simulink model "day10p2"  (R2026a)
settings: Solver=FixedStepDiscrete  StopTime=inf
InitFcn:
  | % lmpCntMax = 6;
  | lmpCntMax = 10;
  | % btnCntMax = 10;
  | btnCntMax = 16;
  | % btnStrMax = 39;
  | btnStrMax = 181;
  | % jltStrMax = 17;
  | jltStrMax = 39;
  | lmpStrMax = lmpCntMax + 2;
  | possibilities = dec2bin([0:((2^btnCntMax) - 1)]) - '0';
  | [~, ixs] = sort(sum(possibilities, 2));
  | possibilities = possibilities(ixs, :);
undefined symbols (not defined in the file): DiscIntNeverNeededParam
libraries: simulink x12
(part 1 of 2)
settings Model: PauseTimes=14  Creator=pete  LastModifiedBy=pete

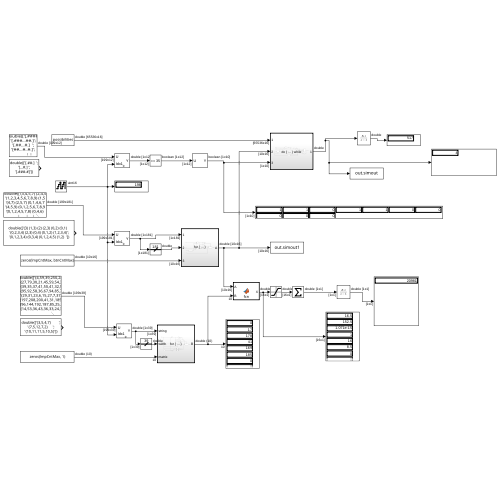
[thumbnail: Simulink's stored preview of the top-level diagram]
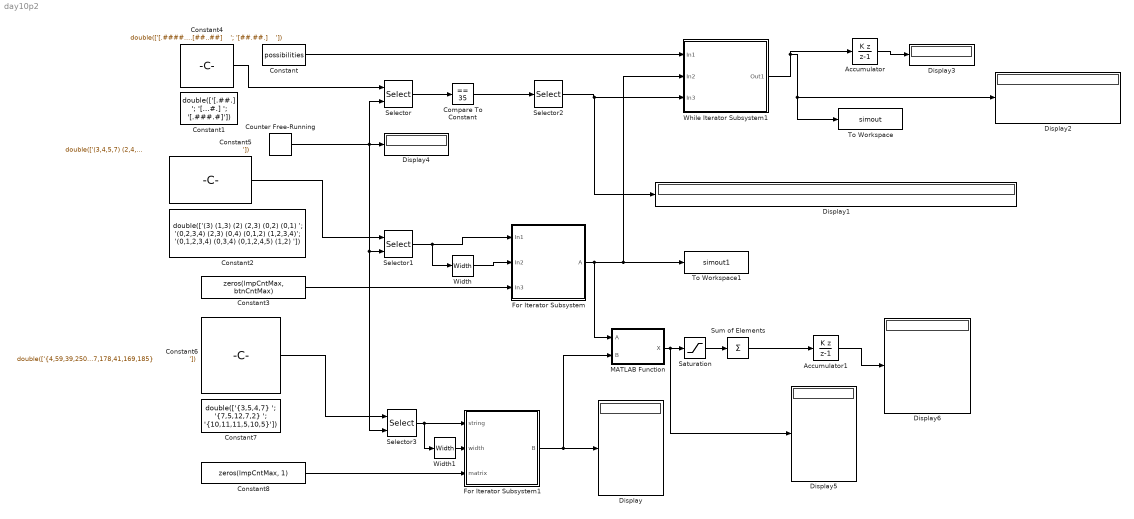
== system day10p2 ==
  Accumulator : DiscreteIntegrator  IntegratorMethod=Accumulation: Backward Euler  SampleTime=-1  ICPrevOutput=DiscIntNeverNeededParam  ICPrevScaledInput=DiscIntNeverNeededParam
  Accumulator1 : DiscreteIntegrator  IntegratorMethod=Accumulation: Backward Euler  SampleTime=-1  ICPrevOutput=DiscIntNeverNeededParam  ICPrevScaledInput=DiscIntNeverNeededParam
  Compare To Constant : simulink/Logic and Bit Operations/Compare To Constant  relop===  const=35  OutDataTypeStr=boolean
  Constant : Constant  Value=possibilities
  Constant1 : Constant  Value=|
      | double(['[.##.]  ';
      | '[...#.] ';
      | '[.###.#]'])
  Constant2 : Constant  Value=|
      | double(['(3) (1,3) (2) (2,3) (0,2) (0,1)        ';
      | '(0,2,3,4) (2,3) (0,4) (0,1,2) (1,2,3,4)';
      | '(0,1,2,3,4) (0,3,4) (0,1,2,4,5) (1,2)  '])
  Constant3 : Constant  Value=zeros(lmpCntMax, btnCntMax)
  Constant4 : Constant  Value=|
      | double(['[.####.#.]  ';
      | '[.###...##.]';
      | '[.##...#.]  ';
      | '[##...#..#.]';
      | '[#...#.#..] ';
      | '[.##...]    ';
      | '[###.....#] ';
      | '[.#.#....]  ';
      | '[###..#..#] ';
      | '[.###]      ';
      | '[...#..#.]  ';
      | '[#.##]      ';
      | '[#####.##.] ';
      | '[.#####]    ';
      | '[.#..###]   ';
      | '[...##.]    ';
      | '[#####.]    ';
      | '[#.##.]     ';
      | '[#....#.##] ';
      | '[.#.#]      ';
      | '[#.#.##.##.]';
      | '[...#]      ';
      | '[..##.#]    ';
      | '[#####.]    ';
      | '[#...#.#]   ';
      | '[##.#..]    ';
      | '[.#..#]     ';
      | '[###.]      ';
      | '[##..#.#..] ';
      | '[###.]      ';
      | '[###.]      ';
      | '[.###]      ';
      | '[##...#.]   ';
      | '[.###.#.]   ';
      | '[#.#...]    ';
      | '[#..##.]    ';
      | '[..##...]   ';
      | '[..#...#]   ';
      | '[.#...##]   ';
      | '[..#..#.#]  ';
      | '[###......] ';
      | '[#.####.]   ';
      | '[..##.##]   ';
      | '[.###]      ';
      | '[.##.#.#..] ';
      | '[#.#.]      ';
      | '[###..#.#]  ';
      | '[#.#..#.]   ';
      | '[#...##]    ';
      | '[...###..]  ';
      | '[####.]     ';
      | '[#...####]  ';
      | '[##.##....#]';
      | '[.#..#]     ';
      | '[#...#....] ';
      | '[.#.....###]';
      | '[..#.#..#]  ';
      | '[#.##..]    ';
      | '[..##...##] ';
      | '[#.#.....#] ';
      | '[.#..##]    ';
      | '[..###]     ';
      | '[.#....#.]  ';
      | '[#.#....###]';
      | '[...#.#.#.] ';
      | '[#..##]     ';
      | '[####]      ';
      | '[..#...##]  ';
      | '[#..#]      ';
      | '[.####.]    ';
      | '[..##.#..##]';
      | '[#.#..##]   ';
      | '[...#..#.]  ';
      | '[#.##...#..]';
      | '[.#..####.#]';
      | '[.#.#]      ';
      | '[##..#.###] ';
      | '[.##.....#.]';
      | '[.....#.#]  ';
      | '[#.#.]      ';
      | '[#.####.###]';
      | '[.##.]      ';
      | '[###..]     ';
      | '[##...#.]   ';
      | '[.#.#.#]    ';
      | '[#...##.]   ';
      | '[###.]      ';
      | '[...#]      ';
      | '[#...#..]   ';
      | '[##..#]     ';
      | '[...#]      ';
      | '[###.]      ';
      | '[#..#####.] ';
      | '[#.#.]      ';
      | '[#...]      ';
      | '[#..##.]    ';
      | '[.#.....]   ';
      | '[###.]      ';
      | '[##...####.]';
      | '[.####.#.#.]';
      | '[.#.##]     ';
      | '[######...] ';
      | '[#..#..#]   ';
      | '[.##...#.]  ';
      | '[...#.#]    ';
      | '[##..#.#.##]';
      | '[....##..]  ';
      | '[####..#.]  ';
      | '[#....#..##]';
      | '[....#]     ';
      | '[.#.#.]     ';
      | '[##...#.#.] ';
      | '[#...#]     ';
      | '[....#]     ';
      | '[###.##..]  ';
      | '[#.#.]      ';
      | '[..#..#]    ';
      | '[#.#.#]     ';
      | '[.#.##]     ';
      | '[.#.#.###..]';
      | '[######..]  ';
      | '[##.##]     ';
      | '[###.##]    ';
      | '[......#..] ';
      | '[##.#.]     ';
      | '[##.#.##..#]';
      | '[.###.]     ';
      | '[..##.###.] ';
      | '[#.#....]   ';
      | '[...#.#..]  ';
      | '[..#.##....]';
      | '[#.##]      ';
      | '[...##]     ';
      | '[#####.#]   ';
      | '[#.##..]    ';
      | '[##..#####] ';
      | '[...##.##.] ';
      | '[.#.#]      ';
      | '[##..]      ';
      | '[.....##..] ';
      | '[###.#..#]  ';
      | '[.##.#.###.]';
      | '[..####]    ';
      | '[#.......##]';
      | '[##.##.]    ';
      | '[###..##]   ';
      | '[####..#.#] ';
      | '[.###..#.#.]';
      | '[.###]      ';
      | '[.....###.#]';
      | '[.###..###.]';
      | '[##.#]      ';
      | '[#.#.]      ';
      | '[.#..#]     ';
      | '[..###]     ';
      | '[.######]   ';
      | '[####...#.] ';
      | '[.#.....#.] ';
      | '[...#.###]  ';
      | '[####]      ';
      | '[#.####..]  ';
      | '[...####]   ';
      | '[#.##.#....]';
      | '[#...###]   ';
      | '[.#.#]      ';
      | '[.##.#.##.] ';
      | '[.##.##.]   ';
      | '[##.#.]     ';
      | '[#.#.]      ';
      | '[#.#.]      ';
      | '[##.###.##.]';
      | '[..##.#.]   ';
      | '[#..##.###.]';
      | '[#......#.] ';
      | '[......#..#]';
      | '[#..#.##]   ';
      | '[...###.]   ';
      | '[..#.#...#.]';
      | '[.#.#.#####]';
      | '[#.#....]   ';
      | '[#.##]      ';
      | '[.#.#.###.#]';
      | '[#.###.]    ';
      | '[#...#.....]';
      | '[.###.##.]  ';
      | '[.....#]    ';
      | '[.####.#..#]';
      | '[.#....]    ';
      | '[.#...]     ';
      | '[#.##.###.#]';
      | '[.###.]     ';
      | '[##.##]     ';
      | '[#.#...##.] ';
      | '[#....##.]  ';
      | '[#.#.###]   ';
      | '[#.##.#..##]';
      | '[##..##.#]  ';
      | '[##..##]    ';
      | '[##.##.]    '])
  Constant5 : Constant  Value=|
      | double(['(3,4,5,7) (2,4,5,6,7) (1,4,7) (1,3,4,7) (1,2,3,4,5,7) (7) (1,2,3,6) (0,1,3,6,7)                                                                                                      ';
      | '(1,2,3,4,5,6,7,8,9) (1,5) (0,1,3,4,5,6,7,8,9) (4,8,9) (0,6,7,9) (1,6,8) (0,1,2,5,6,7,8) (0,1,2,3,5,7,8,9) (1,2,4,5)                                                                  ';
      | '(4,7) (2,5,7) (0,1,4,6,7) (1,4) (0,3,4,5,6,7) (0,1,2,3,4,5,7) (0,1,2,3,4,6) (2,3,5,6,7)                                                                                              ';
      | '(4,5,9) (0,1,2,5,6,7,8,9) (0,1,4,5,6,7,9) (0,1,2,5,6,8) (0,1,2,3,5,7) (1,2,3,4,5,6,8,9) (0,1,3,4,5,6,7,8,9) (3,4,8) (0,4,7,9)                                                        ';
      | '(0,1,2,4,5,7,8) (0,4,6) (0,1,2,7,8) (1,7,8) (1,2,3) (0,5,7,8) (0,1,4,5,6,7) (1,2,5,7,8)                                                                                              ';
      | '(1,3,4) (0,1,3) (3,5) (0) (0,1,2,5) (2,3,4)                                                                                                                                          ';
      | '(0,1,2,3,4,8) (0,3,4,7) (0,1,2,4,5,6,7) (2,3,4) (0,4) (1,2,3,7,8) (0,2,3,6,8) (0,2,4,5,7) (0,1,4,5,6,7,8)                                                                            ';
      | '(1,2,3,4,5,6,7) (1,3) (1,2,3,4,5,7) (1,7) (0,1,2,3,4,6,7) (0,2,4,5,6)                                                                                                                ';
      | '(1,4,5,6) (0,3,7) (1,6,7) (1,2,3,4,8) (0,4,7) (3,4,7) (2,3,5,8)                                                                                                                      ';
      | '(3) (0) (1,3) (1,2) (0,2,3)                                                                                                                                                          ';
      | '(0,2,3,5,6) (1,3,5,6) (5,7) (0,4,7) (1,7) (0,1) (2,4) (0,2,3,4,5,6) (0,3,4,5,6,7) (0)                                                                                                ';
      | '(1,3) (0,3) (0,2,3)                                                                                                                                                                  ';
      | '(1,5,8) (1,2,3,5,6) (2,4,8) (3,4,8) (2,4) (0,1,7,8) (2,3,6) (2,3,7,8) (4,7)                                                                                                          ';
      | '(0,1,3) (0,2) (0,3,4,5) (0,1,4) (0,4)                                                                                                                                                ';
      | '(0,1,4) (1,2) (1,2,3,4,5,6) (0,3,5) (2,3)                                                                                                                                            ';
      | '(2,5) (3) (1,4) (0,1) (0,1,4,5) (4) (2,4,5) (1,2,3,4)                                                                                                                                ';
      | '(0,1,3,4,5) (1,2,3,4) (3) (3,5) (1,5) (0,1,2,4) (2,5) (0,1,2,3)                                                                                                                      ';
      | '(0,1,3,4) (0,1,3) (0,2,3)                                                                                                                                                            ';
      | '(4) (2,3,7) (2,3,4,7,8) (0,1,4,5) (2,3,5,6) (1,2,3,5,6,7,8) (0,3,5,7)                                                                                                                ';
      | '(1,2) (0,2) (0,1,2) (3)                                                                                                                                                              ';
      | '(2,5,6,8) (0,1,2,3,4,5,7,8) (2,7) (0,2,3,6,8) (0,4,6,7,9) (0,1,3,4,5,8,9) (3,4,8) (0,1,5,8)                                                                                          ';
      | '(0,3) (0,2) (1,3) (0,1,3)                                                                                                                                                            ';
      | '(1,3) (0,5) (2,3,4) (0,1,3,4) (1,2,5)                                                                                                                                                ';
      | '(3,4,5) (0,1,2,4,5) (2,3,5) (0,1,5) (1,2,3) (0,2,4,5) (4,5)                                                                                                                          ';
      | '(3,5,6) (0,1,2,5,6) (0,1,2,3,6) (4,6) (2,4,5,6) (0,1,2,3,4) (1,2,3) (0,1,2,4,5) (1,2,3,4,6)                                                                                          ';
      | '(1,2,3,5) (0,3,4,5) (1,2) (0,1,3)                                                                                                                                                    ';
      | '(0,2) (1,4) (0,1,3,4) (0,3,4)                                                                                                                                                        ';
      | '(3) (0) (0,1) (0,1,2) (1,2)                                                                                                                                                          ';
      | '(0,3,4,5,6,7,8) (1,2,4,5,6,7,8) (2,4,7) (0,1,4,6) (1,2,3,4,5,6,7) (1,3,4,5,6) (0,1,3,5,8) (0,1,4,8)                                                                                  ';
      | '(0,1,2) (0,1,3)                                                                                                                                                                      ';
      | '(1,2) (0,2,3) (0,3) (0,1)                                                                                                                                                            ';
      | '(1,2,3) (0,2,3)                                                                                                                                                                      ';
      | '(3,4,6) (1,2,4,5) (0,1,5) (1,6) (0,2,3,5,6)                                                                                                                                          ';
      | '(0,1,2,3,6) (2,3,5,6) (1,2) (3,5) (0,2,4,5,6) (1)                                                                                                                                    ';
      | '(1,4,5) (0,3,4,5) (3,4) (2,5)                                                                                                                                                        ';
      | '(0,1,4,5) (1,2,5) (0,1,2,4) (3,5)                                                                                                                                                    ';
      | '(2,3) (0,1,3,5,6) (2,4) (0,2,3,4,5,6) (0,5)                                                                                                                                          ';
      | '(0,2,6) (1,3) (0,1,2,3,5,6) (1,3,4,5,6) (4,5,6) (1,2,3,4)                                                                                                                            ';
      | '(1,2,4,5) (0,2,3,4,5) (0,2) (0,5) (0,2,4,6) (1,5,6)                                                                                                                                  ';
      | '(1,2,4,7) (1,4,5) (0,1,3,6) (0,1,2,4,6) (2,3,5,7) (0,3,4,5,6,7)                                                                                                                      ';
      | '(0,1,3,4,7) (1,2,3) (1,8) (2,7) (0,1,4,5,7,8) (0,1,3,6,7) (0,1,2,3,4,5,7) (0,1,4,7,8) (0,1,3,4,6,7,8)                                                                                ';
      | '(0,2,3,4,5) (0,1,3,5,6) (0,3,4,5) (0,1,5,6) (2) (1,2,3,4,6) (0,1,3,4,5) (0,1,2,3) (0,6)                                                                                              ';
      | '(2,3) (1,4,5,6) (1,2,3,4,5,6) (0,1,2,5,6) (4,5) (0,1,2,3) (1,4) (0,1,3) (0,5)                                                                                                        ';
      | '(0,1) (2,3) (0,2,3)                                                                                                                                                                  ';
      | '(0,1,4,5,6,7,8) (0,1,3,4,5,6,7) (0,1,2,4,5,7,8) (0,1,2,3,4,6,8) (0,1,3,4,5,7,8) (0,2,3) (5,7)                                                                                        ';
      | '(0,1) (2,3) (1,2) (0,3) (0,2)                                                                                                                                                        ';
      | '(0,1,3,4,6,7) (1,2,3,4,5,7) (0,1,7) (1,4,5,6,7) (0,1,5,7) (5,6,7) (0,4) (1,5) (2,3,4,5) (1,4,7)                                                                                      ';
      | '(1,3,4) (0,1,3) (1,3,4,5,6) (1,2,3,5) (0,2,3,4,5)                                                                                                                                    ';
      | '(0,4,5) (3,4) (0,1,2,3,5) (1,2) (1)                                                                                                                                                  ';
      | '(3,4) (0,2,5,6,7) (0,3,5,6) (0,1,2,3,5,7) (1,2,4,5,7) (0,1,3,4,5) (0,2) (2,6,7) (0,1,4,5,6,7) (2,3,4,5,6,7)                                                                          ';
      | '(4) (0,1,3,4) (2,3,4) (1,2,3) (2) (0,3,4) (2,4)                                                                                                                                      ';
      | '(0,1,3,4) (4,5,6,7) (0,1,2,4,5,6,7) (0) (0,1,2,3,5,7) (0,2,3,7) (1,5) (0,2,3,4,6,7)                                                                                                  ';
      | '(1,5,9) (1,3,5,6,7,8,9) (1,2,4,5,8,9) (1,2,4,5,6,7) (1,3,5,6,7,8) (0,1,2,3,4,5,6,7,9) (0,1,3,4,6,7,8,9) (0,1,5,6,7,9) (2,4,6,7,8)                                                    ';
      | '(0,2,4) (0,2) (0,1,2) (1,4) (2,3,4) (1,2,3,4)                                                                                                                                        ';
      | '(0,1,2,4,8) (0,1,4,5,6,7,8) (3,4,5,6,7,8) (1,3,7,8) (0,2,3,4,8) (2,3) (3,6,7) (0,1,4,5,7) (0,1,5,6) (2,7) (0,6,8)                                                                    ';
      | '(0,1,2,3,5,6,7,8,9) (0,2,3,4,6,7,9) (0,1,2,5,8) (0,1,3,7,8,9) (1,4,5,6,7) (0,1,3,8) (0,1,2,3,5,6,8) (0,1,3,4,5,6,7) (1,2,3,5) (1,3,4,5,6,7,8,9)                                      ';
      | '(0,1,2,3,6) (4,6) (1,2,3,5) (2,3,7) (0,5,6) (0,1,4,6) (0,1,3,5) (1,6,7) (4,7)                                                                                                        ';
      | '(0,1,3,4) (3,4,5) (2,3,4,5) (2,3) (4,5) (1,5)                                                                                                                                        ';
      | '(4,8) (1,4,6,8) (3) (0,1,5) (5,7) (1,2,3,5,7,8) (2,3,4,5) (0) (1,3,4) (0,1,3,4,6,7,8)                                                                                                ';
      | '(6,8) (1,2,3,4,7,8) (1,6,8) (1,2,3,6,7) (1,2,3,5,8) (2,6) (3,4,5,8) (0,2) (1,2,3,4,5,6)                                                                                              ';
      | '(2,4,5) (0,1,3) (4,5) (0,1,5) (0,2,3,4,5)                                                                                                                                            ';
      | '(1,2) (0,1,3) (1,3,4)                                                                                                                                                                ';
      | '(6) (0,4,5) (1,2,4,6) (1,2,3,4,7) (0,1,2,3) (0,1,2,4,5,7) (0,4) (1,7) (0,3,7)                                                                                                        ';
      | '(0,1,2,3,4,5,6,8) (1,3,4,5,7,8,9) (1,2,3,5,6,7,9) (6,8) (6,7) (1,3,5,7,8) (0,1,2,3,6,8,9) (1,2,4,5,6,7,8,9) (0,1,2,3,5,6,8,9) (0,1,4,5,6,7,8,9)                                      ';
      | '(0,1,2,6,7) (0,1,3,4,5,7,8) (1,3,8) (0,1,3,4,6,7,8) (1) (0,2,4,6,7,8) (4) (3,5,7) (0,1,4,8) (1,4,6) (1,2,3,4,7,8)                                                                    ';
      | '(0,1,2,4) (0,3) (0,2,4) (0,2) (1,4)                                                                                                                                                  ';
      | '(0,1,2) (3) (0,3) (0,1,3) (0,1)                                                                                                                                                      ';
      | '(2,3,4,5,6) (0,1,2,3,4,5,7) (0,4,5,6,7) (1,6,7) (0,1,2) (4,5,6,7) (1,3,4,5,6,7)                                                                                                      ';
      | '(0,1) (1,3) (1,2) (3) (0,3) (0,2)                                                                                                                                                    ';
      | '(1,2,4,5) (0,2,3,5) (0,4,5) (0,2)                                                                                                                                                    ';
      | '(2,3,4,5,9) (2,3,4,6,8,9) (0,1,2,3,5,6,7,9) (3,5,6,9) (0,8) (0,3,4,5,6,9) (0,4,8) (1,3,7,8) (1,4,5,7,8) (0,3,4,5) (0,2,3,4,6,7)                                                      ';
      | '(1,2,4,6) (2,5,6) (3,4) (1,3,4,5,6) (0,1,2,4,6) (0,5) (0,1,2,5)                                                                                                                      ';
      | '(1,2,3) (1,4) (0,1,3,4,5,7) (0,7) (1,5) (1,7) (0,2,4,5,6,7) (0,4) (3) (4,5)                                                                                                          ';
      | '(1,2,6,7) (0) (3,4) (0,1,2,5,7,8,9) (7,8) (0,1,2,3,4,6,7,8,9) (6,7,9) (1,2,4,5,7) (0,3,7) (1,3,4,5,6,7,8,9) (1,3,4,6,7,8,9) (0,1,2,4,6)                                              ';
      | '(0,5,7,8) (2,3,4,8,9) (1,2,3,5,8) (0,1,3,4,5,7,8,9) (4,5,6,7,8) (0,2,3,5,8,9) (1,2) (0,1,2,3,6,8) (0,2,4,5,8)                                                                        ';
      | '(1,2) (0,1,3) (2,3)                                                                                                                                                                  ';
      | '(0,2,3,6,7,8) (1,2,5,7) (0,1,2,3,6,7) (2) (0,4,5,8) (1,3,6,7,8) (1,4,5,7,8) (0,2,4,5,6,7) (0,1,2,4,6,7,8) (1,3,5) (1,4,6)                                                            ';
      | '(0,3,7,9) (2,7) (0,2,9) (2,3,8,9) (1,2,3,4,5,7,8,9) (4,7,8) (0,1,3,5,6,7,8) (5,8) (0,2,4,5,6,7,8) (1,7)                                                                              ';
      | '(0,5,7) (0,1,3,4,5,6) (0,1,2,3,6,7) (0,1,2,3) (1,3,4,6,7) (0,4,7) (0) (0,1,3,5,6,7) (1,3,4)                                                                                          ';
      | '(2,3) (0,1,2) (0,2) (0,1) (2)                                                                                                                                                        ';
      | '(0,8,9) (0,2,4,5,6,8,9) (3,4,6,9) (0,1,4,5,6,7,8,9) (1,3,8) (0,2,3,4,5,7,8,9) (0,2,3,6,7) (0,1,2,4,5,6,7,8) (1,6,8)                                                                  ';
      | '(0,3) (2,3) (1,3) (2)                                                                                                                                                                ';
      | '(4) (1) (3,4) (2,3,4) (0,2,3) (0,2)                                                                                                                                                  ';
      | '(0,3) (2,4,5) (0,1,2,4) (0,5,6) (0,2,4,5,6) (1,4,6) (1,2,3)                                                                                                                          ';
      | '(1,4,5) (1,2) (3,4) (0,4,5) (0,2,4) (2,5)                                                                                                                                            ';
      | '(1,2,3,4) (1,2,3,5) (5,6) (4) (0,1,6) (1,3,5,6) (0,2,3,5) (3) (1)                                                                                                                    ';
      | '(0) (0,2,3) (0,1,3) (1,3)                                                                                                                                                            ';
      | '(0,2) (0,1,3) (0,3) (2,3) (1,3) (1,2,3)                                                                                                                                              ';
      | '(4,6) (2,3) (0,2,3,4,5,6) (0,1,2,5) (4,5,6) (1,2,3,5,6) (0,1,3,4,6) (2,3,4,5)                                                                                                        ';
      | '(0,1,2,3) (4) (2,3) (0,3,4) (0,1,4) (0,1) (1,3)                                                                                                                                      ';
      | '(1,2,3) (1) (0,3) (0,2,3) (2)                                                                                                                                                        ';
      | '(0,3) (3) (0,1,2) (0,1) (2,3) (0,2)                                                                                                                                                  ';
      | '(1,2,3,5,6,7,8) (1,3,8) (5,7) (0,1,2,3,4,6,7) (0,1,2,6,7,8) (0,2,3,4,5) (2,3) (1,2,5) (0,7) (0,7,8)                                                                                  ';
      | '(1,2,3) (1,2) (0,1,3)                                                                                                                                                                ';
      | '(2,3) (1,2) (0,1) (1,3) (0,2,3)                                                                                                                                                      ';
      | '(0,1,2,4) (1,3,5) (0,1,4) (1,3)                                                                                                                                                      ';
      | '(1) (0,1,3,4) (1,2,3,4,5,6) (1,5) (1,2,4,5,6) (0,1,2,3,4,6) (0,4,5)                                                                                                                  ';
      | '(1,2) (0,1,2) (1,3) (3) (0) (1)                                                                                                                                                      ';
      | '(1,2,5,6,7,8,9) (2,4,9) (3,4,6,7,8,9) (0,5) (0,1,2,7,9) (0,1,4,5,7,9) (1,3,8) (1,2,3,4,5,6,8,9) (1,2,3,4,6,8,9) (0,1,2,3,4,5,7,8,9) (0,1,3,4,5,6,7) (1,2,4,5,6,7,9) (0,1,2,3,4,5,8,9)';
      | '(0,1,2,4,5,6,7,8) (7,9) (1,2,3,4,5,6,7,8,9) (0,4,5,8) (5) (2,5) (2,3,9) (0,1,3,4,6,7,8) (7,8,9) (3,4) (0,1,3,5,7,8) (1,6,7) (0,1,2,3,4,5,6,8)                                        ';
      | '(0,2) (0,1,2,4) (0,2,3)                                                                                                                                                              ';
      | '(3,4,5) (0,2,4) (0,1,2,3,5,7,8) (2,3) (1,8) (0,1,4,5,6,7,8) (0,4,5,6) (1,2,3,5,6,7,8) (3,4,7) (1,2,4,5,6,7)                                                                          ';
      | '(0,1,2,3,4,5) (0,1,3) (0,6) (0,4) (0,1,2,4,5) (1,2,3,4,5)                                                                                                                            ';
      | '(0,1,3,4,5,6,7) (1,2,5,6) (0,3,6) (0,6,7) (1,2,4,5,7) (2,3,5,6) (1,2,4,7)                                                                                                            ';
      | '(1,5) (1,3,4,5) (2,3,4,5) (0,1,2,3) (4) (2,3)                                                                                                                                        ';
      | '(1,3,4,5,6,7,9) (0,7) (0,1,2,3,6,8,9) (0,1,4,5,7,8,9) (4,5) (3,4,8) (0,1,3,6,8) (0,2,3,4,5,6,7) (1,3,8) (0,1,2,4,5,7,8,9)                                                            ';
      | '(2,3,4,5) (4,5) (1,2,3,4,5,7) (1,2,7) (0,1,2,3) (0,1,3,4,6)                                                                                                                          ';
      | '(0,1,3,6) (0,1,2,5,6) (1,5) (0,3,5,6,7) (0,3,4,6,7) (1,2,3,4,6,7) (0,1,2,3,6,7)                                                                                                      ';
      | '(0,1,3,5,7,8) (1,2,3,6,9) (2,4,5,7,8) (0,1,2,6,7,8,9) (0,5,7) (1,2,6,7) (1,4) (5,8) (3) (4,5,7,8,9) (3,6)                                                                            ';
      | '(0,1,3) (2,3) (0,1,3,4)                                                                                                                                                              ';
      | '(0,4) (1,4) (0,2,4) (3,4)                                                                                                                                                            ';
      | '(0,1,4,5,6,8) (0,1,2,3,6,8) (0,4,5,6,7) (0,2,3,4,7) (0,2,3,6,8) (0,1,2,5,6,7,8) (1,3,7) (1,2,6)                                                                                      ';
      | '(0,1,3) (2,3) (1,3,4)                                                                                                                                                                ';
      | '(2,3,4) (0,1,3) (0,2) (2) (1,2,3) (3,4) (0,1,2)                                                                                                                                      ';
      | '(0,1,2,4,7) (2,3) (1,3,5,7) (0,1,2,3,7) (0,3,4,6) (0,1,7) (0,1,2,5,6,7) (0,1,2,7) (5,7) (2,6,7)                                                                                      ';
      | '(1,2,3) (0,2)                                                                                                                                                                        ';
      | '(2,3,5) (0,1,3,4) (2,5) (1,3,5) (1,5) (0,2) (0,2,3,5)                                                                                                                                ';
      | '(1,2) (3) (1) (4) (1,3,4) (0,2) (0,2,4)                                                                                                                                              ';
      | '(2,3) (0,2) (0,3,4) (0,1,2,3) (0,1,2)                                                                                                                                                ';
      | '(0,3,4,5,6,7,9) (1,2,4,5,6,7,8) (4,5) (0,1,2,4,5,6,7,8) (0,1,4,5,6,8) (0,3,4,5,7,8,9) (1,6) (5,6,8) (1,4,6,8,9) (0,1,6) (0,1,2,4,5,7,8,9)                                            ';
      | '(1,2,3,5,6,7) (0,1,3,6) (5,6) (0,2,3,7) (0,1,3,4,5) (0,1,2,3,4,5) (2,3,4,5,6) (0,1,2,4,5)                                                                                            ';
      | '(0,1,2,3) (2,4) (0,1,2) (0,2,4) (1,3)                                                                                                                                                ';
      | '(0,2,3,4,5) (1,5) (0,1) (0,2,4) (2,3,4,5) (0,3,5) (0,3)                                                                                                                              ';
      | '(0,2,3,4,6,7,8) (0,1,2,3,4,6,7) (1) (0,3,4,5,6,7) (0,1,2,3,4,5,6,8) (3,4,7) (0,1,2,3,5,7,8) (4,6,7) (5,6,7) (4,5,6,8) (1,4,6,7)                                                      ';
      | '(0,1,4) (1,3,4) (0,1,2) (0,3) (0,2)                                                                                                                                                  ';
      | '(0,1,4,5,6,7,8,9) (0,2,4,5,6,7,8,9) (1,3,5,8) (0,2,5,9) (2,4,6,7,8) (1,5,9) (2,4,5,6,9) (0,2,4,8) (0,2,3,4,5,7,8,9) (0,1,2,3,4,5,6,7) (1,2,4,5,7,8,9) (2,4,7,8,9)                    ';
      | '(1,3,4) (1,2,3,4) (0,1) (2,3,4) (1,2) (0,1,2,4)                                                                                                                                      ';
      | '(0,1,2,3,4,6,7,8) (1,4,8) (0,1,3,5,7,8) (0,2,3,4,6,8) (0,1,2,6,7,8) (2,3,4,5,6) (1,2,3,5,6,7,8)                                                                                      ';
      | '(1,2,5) (0,1,2,5) (0,2,4,5) (1,2,4) (0,3,4) (0,2) (0,3,4,6)                                                                                                                          ';
      | '(1,4,5,6,7) (3,4) (0,1,2,3,6,7) (1,2,3,4,7) (0,2) (3,5) (3,4,6) (0,1,2,4,5,7)                                                                                                        ';
      | '(0,3,6,9) (4,8) (0,1,3,4,5,6,7,8) (2,8,9) (1,2,3,4,5,6,9) (2,3,4,6,7,8) (3,5,6,7) (0,2,3,5,7,9) (0,1,5) (0,1,5,6,8,9) (2,4,5,8,9) (1,2,3,5,6,7) (0,2,3,5,6,7,8,9)                    ';
      | '(0,2,3) (0,1,3)                                                                                                                                                                      ';
      | '(2,4) (0,1,4) (0,1,3)                                                                                                                                                                ';
      | '(3,4) (1,3,5,6) (1,2) (0,3,4) (5,6) (2,3,4,5,6) (0,1,6) (0,1,2,6)                                                                                                                    ';
      | '(0,2) (1,2,3,4) (1,3) (2,3,5) (0,1,3,4) (0,1,4) (0,2,3,5) (1,3,4,5)                                                                                                                  ';
      | '(0,1,2,4,5,7,8) (0,6,8) (1,2,5,6,8) (0,1,2,3,5) (0,1,4,6,7,8) (4,5,6) (1,3,4,5,7) (1,3,6,7) (2,4,6,7) (1,2,5,6,7,8)                                                                  ';
      | '(1,2,5,6,8) (0,5,8) (3,5,7,8) (3,7) (0,1,2,3,4,5,6,8) (0,4,7) (4,5,6,8) (0,1,2,4,5,7,8)                                                                                              ';
      | '(1,3) (0,2)                                                                                                                                                                          ';
      | '(0,1,3) (2,3) (0,3) (0,2,3) (1)                                                                                                                                                      ';
      | '(0,4,8) (0,1,2,3,5,7) (0,3,4,7) (4,5,6,7,8) (3,5,6) (0,3,6) (0,1,3,4,5,6,7,8) (0,1,5,6) (0,7) (0,3,4,6,7) (0,1,2,4,5,6,8)                                                            ';
      | '(1,2,3) (1,3,5,6,7) (2,4,5) (0,1,4,5,7) (0,2,3,4,5,7) (0,1,2,4,5,6) (0,2,3,5,7)                                                                                                      ';
      | '(0,2,3,7,8,9) (2,3,6,9) (0,1,3,5,7,9) (1,2,3,5,6,7,9) (0,4,5,6,7,8) (2,3,5,6,7) (0,2,3,5,7,9) (1,9) (0,1,2,3,4,6,7,9) (4,8) (0,1,3,4,5,6,8,9)                                        ';
      | '(1,3) (0,2,3,5) (0,1,2,4) (0,2,4,5) (0,1,2,3) (4,5) (2,4) (2,3,4)                                                                                                                    ';
      | '(0,3,5,8) (3,5,6,7,9) (0,2,3,4,5,7,8,9) (5,6,7,9) (1,2,3,4,6,7,8,9) (1,3,4,5,7) (2,4,6,7,8,9) (4,6,8,9) (2,5,6) (2,4,5,6,7,9) (1,2,5,8,9)                                            ';
      | '(0,1,2,4,5) (3,5) (0,1,2,5) (1,2,4,5) (0,1,3,4) (0,3,5) (1,4,5)                                                                                                                      ';
      | '(5) (1,2,4,5) (1,2,4,6) (0,2,4) (0,1,2,3,4,6) (0,1,3,5,6) (0,3,4)                                                                                                                    ';
      | '(0,3,4,6,7) (0,2,4,6) (0,1,2,3,6,8) (1,3,4,5,6,7,8) (1,2,8) (2,3) (5,6,8)                                                                                                            ';
      | '(4,5) (5,7) (0,5,6,8,9) (0,1,5,6,9) (0,1,2,4,5,6,7,8) (3,4) (0,1,3,4,6,7,8,9) (1,4,5,6,7,8,9)                                                                                        ';
      | '(0,2) (1,2,3)                                                                                                                                                                        ';
      | '(8) (1,3,4,6,7,9) (0) (1,2,4,5,6,7,8) (0,1,2,3,6,7) (2,4) (1,5) (1,2,6,8,9) (5,7) (0,2,4,5,8) (0,1,2,3,4,6,7,9) (1,2,3,5,7,8,9)                                                      ';
      | '(9) (0,1,2,6,8) (2,3,6,7,8) (0,5) (0,1,3,5,6,7,8,9) (2,3,4) (1,2,4,5,6,8,9) (2,4,5,7,8) (1,3,5,6,7,8,9) (4,6,9) (0,7) (1,9) (1,2,3,6,8)                                              ';
      | '(1,3) (0,1,3) (1,2)                                                                                                                                                                  ';
      | '(0,2) (1,3) (1) (0,2,3)                                                                                                                                                              ';
      | '(2) (0,1,2,3) (1,4) (0,2,3,4)                                                                                                                                                        ';
      | '(1,2,4) (0,2,4) (1,4) (1,2,3,4) (2,3,4) (0,2,3,4)                                                                                                                                    ';
      | '(1,2,3,4,5) (0,1,3,4,6) (1,2,4,5,6) (0,1,5,6) (0,3) (1,5,6) (0,2) (0,1,2,5,6)                                                                                                        ';
      | '(0,1,2,4,5) (1,2,3,8) (0,2,3,7,8) (0,1,2,3,4,7) (0,1,3,4,6,7,8) (0,2,4,7,8) (0,1,2,3,8) (1,3,5,6,8) (1,2,3,4,5) (0,4,5,7) (2,8)                                                      ';
      | '(0,1,4) (0,1,2,3,4,6,7,8) (3,4,5,6,7) (0,2) (0,2,3,8) (2,3,5,7) (0,1,4,5,7) (0,2,3,4,5,6,7,8)                                                                                        ';
      | '(0,1,2,3,6,7) (3,6,7) (0,3,7) (3,4) (2,3,4,6,7) (0,1,5,6) (1,2,3,4,6) (1,4,5) (0,2,5,6)                                                                                              ';
      | '(0,2) (0,3) (1,3)                                                                                                                                                                    ';
      | '(0,1,3,4,5,6) (1,2,3,5) (0,1,3,5,7) (0,1,2,4,5,6) (1,2,6,7) (1,2,3,4,5,6)                                                                                                            ';
      | '(1,2,3,5,6) (0,3) (4,5) (0,3,6) (0,1,2) (0,3,5) (1,2,4,6) (3,4,6)                                                                                                                    ';
      | '(0,1,2,3,5,6,7,9) (0,4,5,6,8,9) (4,5,6,7) (0,2,3,4,5,6,8) (2,3,4,5,6,9) (0,1,2,4,5,7,8,9) (0,3,4,5,6,8,9) (1,3,6,7,8) (4,6,8) (5,7) (5) (7,8,9)                                      ';
      | '(0,1,3,4,6) (0,2,3,5,6) (2,3,4,6) (1,6) (1,2,3,5,6) (0,6) (2,6)                                                                                                                      ';
      | '(1,3) (0,2,3)                                                                                                                                                                        ';
      | '(2,8) (0,3,4,5,6,7) (1,5,7) (1,2,3,4,6,7,8) (0,1,5,6,7,8) (7) (1,2,3,5,7,8) (2,3,4,6,8) (0,1,2,3,4,7,8) (1,3,4,6,7)                                                                  ';
      | '(0,2,4,5) (1,3,4) (0,1,3,6) (1,2,3,5,6) (1,2,5)                                                                                                                                      ';
      | '(0,3,4) (1,2,4) (0,1,3,4) (2)                                                                                                                                                        ';
      | '(0,2) (0,1,3) (0,2,3) (1,3) (0,3)                                                                                                                                                    ';
      | '(1,3) (0,2)                                                                                                                                                                          ';
      | '(0,1,2,3,4,5,6,9) (0,1,2,4,5,7,8,9) (0,1,7,8) (1,2,3,4,6,7,8,9) (2,3,4,9) (0,1,2,4,6,7,8) (0,1,2,6,9) (3,4,6,7,9)                                                                    ';
      | '(0,4,6) (1,3,6) (1,2,3,5,6) (2,4,5,6) (0,1) (0,2,3,5) (2,3,5)                                                                                                                        ';
      | '(0,1,2,3,4,5,7,8) (4,6) (1,4,5,8) (0,2,3,5,6,7,8,9) (0,3,4,5,7,9) (0,2,5,6) (2,4) (1,9) (0,1,2,3,4,5,7,8,9) (0,1,3,4,6,7,8,9)                                                        ';
      | '(0,3) (0,2,5,6,7) (0,1,3,4,5) (1,2,8) (0,2,3,5,6,7,8) (2,3,6,7) (0,1,2,4,5,6,7,8) (0,2,3,4,5,7,8)                                                                                    ';
      | '(6,9) (1,2,4,5) (0,1,2,3,4,5,6,7,9) (1,2,4,5,7,8,9) (1,3,4,5,7,8) (0,5,6) (1,2,4,5,6,7,8) (0,1,3,4,6,7,8,9) (0,2,3,7,8,9) (3,4,5,6) (1,2,3)                                          ';
      | '(2) (2,4) (0,1,2,3,6) (4,5) (3,6) (3) (0,5) (0,1,3,4,6) (0,2,3,6)                                                                                                                    ';
      | '(1,6) (0,6) (1,2,3,5) (3,4,5) (0,1,2,5,6) (0,2,3,4,5)                                                                                                                                ';
      | '(0,1,2,3,4,5,6,8,9) (1,2,3,4,5,6,7) (1,6,7,8) (4,6) (3,7,9) (0,1,2,3,5,6,9) (2,3,4,7,8) (0,2,4,6,7,8,9)                                                                              ';
      | '(1,2,3,8) (0,3,4,5,6,7,8,9) (2,3,6,7,9) (1,3,4,6,7) (1,5,6) (4,5,8,9) (9) (1,3,4,6,8,9) (1,2,3,6,7,8) (4,5,6,7) (1,2,4,6,8,9) (0,1,7,9)                                              ';
      | '(3) (0,2,3,4,5) (0,2,5) (0,1,2,3,4) (0,1,2,4,5) (0,1,2,3,4,5) (0,1,2,5) (0,2,3,5,6) (3,5)                                                                                            ';
      | '(2) (3) (0) (1) (0,3) (2,3)                                                                                                                                                          ';
      | '(0,1,2,3,4,7,8,9) (0,1,3,4,5,6,8,9) (0,1,3,4,5,6,7,8) (0,1,2,3,4,5,6,8) (0,1,6,7,8,9) (2,7,9) (0,1,3,5,9) (2,5,7,8,9) (1,3,5,6,7,9) (8,9) (3,7) (7)                                  ';
      | '(1,2,3,5) (2) (0,2,3,4) (1,2,3,4) (2,5) (1,2,4,5) (1,3,4) (1,4)                                                                                                                      ';
      | '(0,1,2,3,6,8,9) (1,2,3,6) (1,2,3,4,5,8) (1,2,3,5,6,9) (1,3,4,5,6,7) (2,3,4,5,7,8,9) (0,2,3,5,7,8,9) (0,1,2,4,5,7,8,9) (0,1,3,4,5,6,7,9) (6,7,8) (0,3,4,5,6,7,8,9) (0,2,5,8,9) (3,6)  ';
      | '(0,1,2,3,5,6) (0,1,2,3,4,6) (0,4,6) (0,7) (2,3,4,6,7) (0,5) (0,2,3,4,5,6) (1,3,4,7) (0,2,5) (0,1,2,3,6,7)                                                                            ';
      | '(2,4,5) (2,4) (0,2,3) (1,3) (1,3,4,5) (0,1) (0,2,3,5)                                                                                                                                ';
      | '(3,4,5,7) (0,1,2,5,6,8) (0,2,4,5) (0,2,4,7) (0,1,4,6,7,8,9) (0,1,2,3,4,6,8) (0,1,2,3,5,6,8) (0,2,3,5) (0,1,2,4,5,6,7) (0,3,4,9)                                                      ';
      | '(4,5) (0,2,3) (0,2,4,5) (1,3) (1,2,3,4)                                                                                                                                              ';
      | '(0,2) (3) (1) (1,3) (0,3) (1,4)                                                                                                                                                      ';
      | '(0,2,3,5,6,7,9) (0,4,5,6,7,8,9) (4,7,9) (4,5,6) (2,5) (0,2,6,9) (0,1,2,3,4,5,6,7) (0,1,6,8,9) (1,3,5,6,7,8,9)                                                                        ';
      | '(1,2) (0,3,4) (1,2,3) (0,4)                                                                                                                                                          ';
      | '(2,3) (2) (0,3,4) (1,2)                                                                                                                                                              ';
      | '(0,1,4,5,7,8) (0,1,3,4,5,7) (1,2,3,6,7,8) (2,4,7) (1,2,4,5,6,7,8) (0,1,2,5,6,8) (1,2,4,5,6,8) (0,1,3,5,6,7,8) (0,3,5)                                                                ';
      | '(0,2,3,4,5,6) (5) (2,3) (1,2,3,4,5) (0,1,2) (0,3,6,7) (1,5) (2,3,5,7) (4,6)                                                                                                          ';
      | '(0,3) (0,1,2,5) (1,2,3) (2,3,6) (1,4,5) (0,2,4,5,6) (1,3,4,5,6)                                                                                                                      ';
      | '(1,4,6,8) (0,1,3,4,8,9) (0,2,3,5,8,9) (1,2,3,4,6,7,8,9) (0,1,2,3,4,5,7,8,9) (2,6,7,8,9) (0,1,2,6,7,8) (1,4,5,9) (1,3,4,5,6,8)                                                        ';
      | '(0,2,5) (1,5) (1,3,4,5,6,7) (2,6) (0,2,3,4,5,6,7) (0,2,7) (3,7) (4,6) (0,2,5,6,7)                                                                                                    ';
      | '(0,3,4) (2) (0,1,2,4) (0,1,2,5) (0,2,3)                                                                                                                                              ';
      | '(3,4,5) (2,4,5) (0,2,4) (1,2) (1,2,3,5) (2,3) (2,3,4,5)                                                                                                                              '])
  Constant6 : Constant  Value=|
      | double(['{4,59,39,250,242,220,26,250}           ';
      | '{27,79,30,21,45,59,54,36,50,43}        ';
      | '{39,35,37,41,50,41,32,59}              ';
      | '{95,92,58,36,67,94,85,76,66,85}        ';
      | '{29,31,23,6,15,27,7,37,37}             ';
      | '{197,208,200,41,31,185}                ';
      | '{96,144,192,187,85,25,25,163,160}      ';
      | '{14,53,36,43,36,33,24,35}              ';
      | '{31,22,11,32,31,8,13,41,11}            ';
      | '{27,22,15,214}                         ';
      | '{67,36,187,49,193,61,49,34}            ';
      | '{16,7,6,23}                            ';
      | '{1,181,199,203,34,180,179,12,45}       ';
      | '{169,18,8,154,145,138}                 ';
      | '{25,44,31,27,28,27,15}                 ';
      | '{9,179,182,175,197,17}                 ';
      | '{3,34,20,46,23,25}                     ';
      | '{26,17,9,26,15}                        ';
      | '{24,25,41,53,28,49,25,41,19}           ';
      | '{4,12,14,3}                            ';
      | '{51,31,57,29,31,48,37,42,62,15}        ';
      | '{33,12,12,27}                          ';
      | '{120,125,31,124,124,27}                ';
      | '{25,16,31,24,56,65}                    ';
      | '{214,228,229,233,221,30,46}            ';
      | '{12,30,24,19,6,13}                     ';
      | '{38,18,11,27,34}                       ';
      | '{40,45,26,18}                          ';
      | '{29,46,181,25,200,44,38,189,43}        ';
      | '{34,34,16,18}                          ';
      | '{37,24,26,27}                          ';
      | '{2,20,22,22}                           ';
      | '{25,202,32,23,15,37,208}               ';
      | '{9,32,24,22,3,19,11}                   ';
      | '{9,2,5,12,14,16}                       ';
      | '{7,13,8,11,7,22}                       ';
      | '{40,19,39,53,24,40,38}                 ';
      | '{21,38,36,38,51,37,57}                 ';
      | '{32,28,30,7,30,53,19}                  ';
      | '{28,38,30,26,41,29,28,29}              ';
      | '{79,90,29,62,67,23,26,90,42}           ';
      | '{218,214,27,46,27,203,217}             ';
      | '{54,68,36,54,47,59,26}                 ';
      | '{5,3,2,2}                              ';
      | '{52,47,28,17,47,51,25,51,44}           ';
      | '{41,21,42,32}                          ';
      | '{41,71,25,44,62,72,41,73}              ';
      | '{24,48,15,55,30,29,14}                 ';
      | '{13,28,18,18,19,13}                    ';
      | '{47,41,198,46,42,54,198,211}           ';
      | '{26,16,36,38,59}                       ';
      | '{49,28,39,32,38,32,34,47}              ';
      | '{21,90,49,49,68,71,80,80,76,57}        ';
      | '{15,24,152,137,150}                    ';
      | '{168,159,52,44,171,151,138,166,165}    ';
      | '{68,94,39,99,38,67,60,57,68,43}        ';
      | '{48,68,35,53,11,30,45,23}              ';
      | '{0,1,26,27,23,24}                      ';
      | '{141,169,24,159,142,61,118,140,139}    ';
      | '{8,46,54,40,14,31,35,9,35}             ';
      | '{29,9,34,25,46,50}                     ';
      | '{15,24,6,18,3}                         ';
      | '{79,54,47,40,49,29,20,45}              ';
      | '{16,45,16,32,31,45,200,213,36,39}      ';
      | '{144,182,5,37,178,21,31,34,152}        ';
      | '{150,15,134,16,27}                     ';
      | '{13,8,0,19}                            ';
      | '{42,43,36,25,40,40,28,42}              ';
      | '{18,8,22,7}                            ';
      | '{22,16,35,19,19,38}                    ';
      | '{48,17,205,254,252,66,210,20,219,223}  ';
      | '{23,33,31,17,38,27,31}                 ';
      | '{50,63,28,215,74,48,12,35}             ';
      | '{59,55,54,22,33,12,46,54,24,24}        ';
      | '{51,220,237,76,38,63,17,28,87,51}      ';
      | '{20,21,21,40}                          ';
      | '{30,20,30,10,29,29,18,20,28}           ';
      | '{33,48,39,55,27,42,21,72,77,42}        ';
      | '{251,73,29,73,226,25,42,235}           ';
      | '{22,22,17,3}                           ';
      | '{194,152,168,56,168,163,169,164,198,62}';
      | '{0,18,11,28}                           ';
      | '{4,13,7,22,22}                         ';
      | '{38,22,50,32,31,41,26}                 ';
      | '{30,15,41,8,46,44}                     ';
      | '{166,221,37,62,30,48,182}              ';
      | '{44,28,19,47}                          ';
      | '{13,32,22,42}                          ';
      | '{54,54,55,58,64,72,79}                 ';
      | '{44,37,6,31,38}                        ';
      | '{15,16,25,27}                          ';
      | '{47,34,28,7}                           ';
      | '{64,49,76,47,20,59,33,69,44}           ';
      | '{1,29,28,10}                           ';
      | '{32,49,41,38}                          ';
      | '{15,32,7,17,15,1}                      ';
      | '{44,91,44,41,78,72,44}                 ';
      | '{126,156,143,19}                       ';
      | '{209,264,67,234,249,232,234,233,59,84} ';
      | '{44,41,47,242,227,67,28,64,67,50}      ';
      | '{149,3,149,1,3}                        ';
      | '{36,155,136,54,176,174,155,159,46}     ';
      | '{51,42,29,28,30,29,20}                 ';
      | '{37,40,30,38,29,38,55,35}              ';
      | '{17,42,44,61,50,42}                    ';
      | '{29,36,19,44,68,49,23,44,38,33}        ';
      | '{192,223,52,220,221,38,183,31}         ';
      | '{192,58,36,209,187,25,211,206}         ';
      | '{34,63,49,39,27,42,41,55,51,28}        ';
      | '{23,23,140,163,13}                     ';
      | '{31,17,12,1,49}                        ';
      | '{63,53,45,43,41,35,66,49,33}           ';
      | '{144,160,9,169,16}                     ';
      | '{47,27,53,17,7}                        ';
      | '{78,63,61,41,35,31,43,86}              ';
      | '{7,10,17,10}                           ';
      | '{37,37,36,52,8,56}                     ';
      | '{6,31,11,37,40}                        ';
      | '{33,12,38,21,3}                        ';
      | '{70,65,18,20,74,79,83,38,45,35}        ';
      | '{80,68,61,69,59,68,24,20}              ';
      | '{42,30,58,18,35}                       ';
      | '{60,22,32,37,32,46}                    ';
      | '{54,53,36,57,75,43,84,88,30}           ';
      | '{61,47,26,34,33}                       ';
      | '{57,43,75,27,86,89,41,59,79,84}        ';
      | '{33,78,54,44,64}                       ';
      | '{45,61,52,48,14,37,52,60,66}           ';
      | '{42,39,51,10,22,39,7}                  ';
      | '{11,33,27,49,58,22,23,33}              ';
      | '{53,36,77,93,48,74,81,65,59,69}        ';
      | '{18,1,17,18}                           ';
      | '{13,13,19,7,25}                        ';
      | '{32,46,27,51,32,39,57}                 ';
      | '{31,51,31,70,47,37}                    ';
      | '{22,31,32,13,37,30,63,36,31}           ';
      | '{35,29,29,35,25,53,29,31,53}           ';
      | '{12,15,12,15}                          ';
      | '{137,24,113,150}                       ';
      | '{79,36,29,159,48,173,166,57,48}        ';
      | '{49,178,58,175,66,219,163,186}         ';
      | '{48,43,212,221,43,37,208,57,52,233}    ';
      | '{39,35,42,43,38,40}                    ';
      | '{10,39,64,53,66,84,87,81,57,97}        ';
      | '{35,55,15,43,53,58}                    ';
      | '{36,23,39,20,44,8,19}                  ';
      | '{44,30,58,56,48,14,58,30,34}           ';
      | '{50,49,13,39,68,60,50,45,33,37}        ';
      | '{10,5,15,5}                            ';
      | '{56,71,69,41,42,57,54,65,54,33}        ';
      | '{13,198,37,182,23,175,187,173,188,200} ';
      | '{132,156,13,143}                       ';
      | '{20,20,20,21}                          ';
      | '{37,25,41,37,28}                       ';
      | '{21,173,55,27,199}                     ';
      | '{26,50,46,24,36,46,35}                 ';
      | '{79,112,108,105,73,50,29,50,93}        ';
      | '{59,31,58,47,41,41,24,55,22}           ';
      | '{56,43,36,69,28,26,62,47}              ';
      | '{140,15,123,32}                        ';
      | '{37,83,52,57,32,63,52,38}              ';
      | '{19,21,21,27,11,21,25}                 ';
      | '{223,30,220,207,247,265,237,75,247,70} ';
      | '{33,25,34,39,10,29,57}                 ';
      | '{6,0,6,6}                              ';
      | '{33,50,43,60,47,52,60,71,56}           ';
      | '{16,18,20,14,12,20,12}                 ';
      | '{25,22,30,25,37}                       ';
      | '{53,27,23,47}                          ';
      | '{130,11,130,11}                        ';
      | '{192,205,215,194,220,167,203,62,42,228}';
      | '{27,40,42,31,24,42,48}                 ';
      | '{85,62,60,70,99,89,54,70,67,56}        ';
      | '{184,40,181,192,160,167,39,170,161}    ';
      | '{51,219,199,197,90,83,89,79,61,67}     ';
      | '{28,11,34,182,16,6,175}                ';
      | '{40,23,39,41,35,54,24}                 ';
      | '{30,17,49,49,64,13,53,57,49,47}        ';
      | '{29,88,45,47,54,54,83,64,64,75}        ';
      | '{176,55,176,158,167,160,0}             ';
      | '{23,13,26,41}                          ';
      | '{56,60,59,60,49,58,37,237,71,73}       ';
      | '{19,52,66,51,63,27}                    ';
      | '{50,57,75,78,55,95,55,80,68,85}        ';
      | '{76,46,205,204,176,48,186,189}         ';
      | '{29,38,45,59,39,53}                    ';
      | '{113,64,81,75,89,72,64,39,49,32}       ';
      | '{15,12,15,21,13,13}                    ';
      | '{2,16,2,19,13}                         ';
      | '{82,38,65,44,57,91,109,66,38,79}       ';
      | '{4,199,199,198,4}                      ';
      | '{18,9,10,19,18}                        ';
      | '{80,99,70,57,72,105,67,79,82}          ';
      | '{24,43,57,44,34,52,18,0}               ';
      | '{33,45,41,22,31,49,22}                 ';
      | '{23,42,43,33,42,36,30,31,53,63}        ';
      | '{211,19,229,18,28,60,60,202}           ';
      | '{152,128,166,24,7,127}                 ';
      | '{0,17,178,41,169,185}                  '])
  Constant7 : Constant  Value=|
      | double(['{3,5,4,7}        ';
      | '{7,5,12,7,2}     ';
      | '{10,11,11,5,10,5}'])
  Constant8 : Constant  Value=zeros(lmpCntMax, 1)
  Counter Free-Running : simulink/Sources/Counter Free-Running  NumBits=16  tsamp=-1
  Display{,1..6} (7 alike) : Display
  For Iterator Subsystem : Subsystem  TreatAsAtomicUnit=on
  For Iterator Subsystem1 : Subsystem  TreatAsAtomicUnit=on
  MATLAB Function : MATLAB Function  TreatAsAtomicUnit=on
  Saturation : Saturate  UpperLimit=1000  LowerLimit=0
  Selector : Selector  NumberOfDimensions=2  IndexMode=Zero-based  InputPortWidth=3  IndexOptions=Index vector (port),Select all  Indices=[1 3],1  OutputSizes=1,1  RuntimeRangeChecks=on
  Selector1 : Selector  NumberOfDimensions=2  IndexMode=Zero-based  InputPortWidth=3  IndexOptions=Index vector (port),Select all  Indices=[1 3],1  OutputSizes=1,1  RuntimeRangeChecks=on
  Selector2 : Selector  IndexMode=Zero-based  InputPortWidth=lmpStrMax  IndexOptions=Index vector (dialog)  Indices=[1:lmpCntMax]  OutputSizes=1  RuntimeRangeChecks=on
  Selector3 : Selector  NumberOfDimensions=2  IndexMode=Zero-based  InputPortWidth=3  IndexOptions=Index vector (port),Select all  Indices=[1 3],1  OutputSizes=1,1  RuntimeRangeChecks=on
  Sum of Elements : Sum  Inputs=+
  To Workspace : ToWorkspace  VariableName=simout  SaveFormat=Timeseries  SampleTime=-1
  To Workspace1 : ToWorkspace  VariableName=simout1  SaveFormat=Timeseries  SampleTime=-1
  While Iterator Subsystem1 : Subsystem  TreatAsAtomicUnit=on
  Width : Width
  Width1 : Width
  wires:
  Constant4/1 -> Selector/1
  Constant5/1 -> Selector1/1
  Selector/1 -> Compare To Constant/1
  Compare To Constant/1 -> Selector2/1
  Selector1/1 -> Width/1, For Iterator Subsystem/1(In1)
  Width/1 -> For Iterator Subsystem/2(In2)
  For Iterator Subsystem/1(A) -> MATLAB Function/1(A), To Workspace1/1, While Iterator Subsystem1/2(In2)
  Selector2/1 -> Display1/1, While Iterator Subsystem1/3(In3)
  While Iterator Subsystem1/1(Out1) -> Accumulator/1, To Workspace/1, Display2/1
  Constant/1 -> While Iterator Subsystem1/1(In1)
  Accumulator/1 -> Display3/1
  Constant3/1 -> For Iterator Subsystem/3(In3)
  Counter Free-Running/1 -> Selector3/2, Selector1/2, Selector/2, Display4/1
  Constant6/1 -> Selector3/1
  Selector3/1 -> Width1/1, For Iterator Subsystem1/1(string)
  Width1/1 -> For Iterator Subsystem1/2(width)
  Constant8/1 -> For Iterator Subsystem1/3(matrix)
  For Iterator Subsystem1/1(B) -> MATLAB Function/2(B), Display/1
  MATLAB Function/1(X) -> Display5/1, Saturation/1
  Saturation/1 -> Sum of Elements/1
  Accumulator1/1 -> Display6/1
  Sum of Elements/1 -> Accumulator1/1
